simulink model "ss_ulinsys_itae_sim"  (Simulink 5.0)
settings: Solver=ode4  StartTime=0.0  StopTime=30  RelTol=1e-3  AbsTol=1e-6
values from neighbouring files (symbols this model uses):
  a = -0.7962    [ss_rapport_itae.m]    (also in ss_rapport_lqr.m; ss_rapport_lqr_tunet.m)
  b = -27.87    [ss_rapport_itae.m]    (also in ss_rapport_lqr.m; ss_rapport_lqr_tunet.m)
  K_itae_d = acker(sysd.a,sysd.b,pcd_itae)    [ss_rapport_itae.m]    (also in ss_rapport_lqr.m; ss_rapport_lqr_tunet.m)
  loopsysd = c2d(loopsys,Ts)    [ss_rapport_itae.m]    (also in ss_rapport_lqr.m; ss_rapport_lqr_tunet.m)
  Lr = (acker(loopsysd.a(2,2)',loopsysd.a(1,2)',estpoled))'    [ss_rapport_itae.m]    (also in ss_rapport_lqr.m; ss_rapport_lqr_tunet.m)
  Nbar = Nu + K_itae_d*Nx    [ss_rapport_itae.m]    (also in ss_rapport_lqr.m; ss_rapport_lqr_tunet.m = Nu + K_lqr_d*Nx)
  Ts = 1/50    (= 0.02)    [ss_rapport_itae.m]    (also in ss_rapport_lqr.m; ss_rapport_lqr_tunet.m)
undefined symbols (not defined in the file or in its folder): sigbuilder_block
libraries: simulink x1
settings Model: Creator=ubha02  LastModifiedBy=mikkel  ExtModeAutoUpdateStatusClock=off

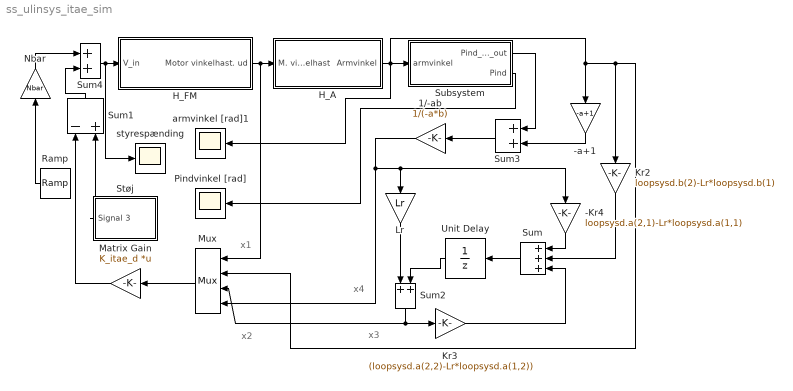
== system ss_ulinsys_itae_sim ==
  note: x4
  note: x3
  note: x2
  note: x1
  -Kr4 : Gain  Orientation=down  Gain=loopsysd.a(2,1)-Lr*loopsysd.a(1,1)  SaturateOnIntegerOverflow=on
  -a+1 : Gain  Orientation=down  Gain=-a+1  SaturateOnIntegerOverflow=on
  1/-ab : Gain  Orientation=left  Gain=1/(-a*b)  SaturateOnIntegerOverflow=on
  H_A : Subsystem
  H_FM : Subsystem
  Kr2 : Gain  Orientation=down  Gain=loopsysd.b(2)-Lr*loopsysd.b(1)  SaturateOnIntegerOverflow=on
  Kr3 : Gain  Gain=(loopsysd.a(2,2)-Lr*loopsysd.a(1,2))  SaturateOnIntegerOverflow=on
  Lr : Gain  Orientation=down  Gain=Lr  SaturateOnIntegerOverflow=on
  "Matrix Gain " : Gain  Orientation=left  Gain=K_itae_d  Multiplication=Matrix(K*u)  SaturateOnIntegerOverflow=on
  Mux : Mux  Orientation=left
  Nbar : Gain  Orientation=up  Gain=Nbar  SaturateOnIntegerOverflow=on
  Pindvinkel [rad] : Scope
      settings: SaveName=pindvinkel  DataFormat=Array
  Ramp : simulink/Sources/Ramp  Orientation=left  slope=0.02  start=0  X0=0
  Støj : Subsystem  Tag=STV Subsys  Orientation=left  StartFcn=sigbuilder_block('start');  StopFcn=sigbuilder_block('stop');  ClipboardFcn=sigbuilder_block('clipboard');  mask(Sigbuilder block){}
      mask help: Sigbuilder GUI
      mask init:
      | if ~strcmp(get_param(bdroot,'SimulationStatus'),'stopped') tuvar = sigbuilder_block('maskInit'); end
      settings: CopyFcn=sigbuilder_block('copy');  DeleteFcn=sigbuilder_block('delete');  ModelCloseFcn=sigbuilder_block('modelClose');  PreSaveFcn=sigbuilder_block('preSave');  NameChangeFcn=sigbuilder_block('namechange');  OpenFcn=sigbuilder_block('open',[50 50 520 400 ]);  CloseFcn=sigbuilder_block('close');
      mask Display: plot(0,0,100,100,[10,10,40,40,10],[80,20,20,80,80],[40,10],[50,50], [40,27,10],[65,72,56],[40,25,25,10],[28,28,43,43]);
  Subsystem : Subsystem
  Sum : Sum  Orientation=left  Inputs=+++  SaturateOnIntegerOverflow=on
  Sum1 : Sum  Orientation=up  Inputs=-+  SaturateOnIntegerOverflow=on
  Sum2 : Sum  Orientation=down  SaturateOnIntegerOverflow=on
  Sum3 : Sum  Orientation=left  SaturateOnIntegerOverflow=on
  Sum4 : Sum  SaturateOnIntegerOverflow=on
  Unit Delay : UnitDelay  Orientation=left  SampleTime=Ts
  armvinkel [rad]1 : Scope
      settings: SaveName=armvinkel  DataFormat=Array
  styrespænding : Scope
      settings: SaveName=styrespaending  DataFormat=Array
  wires:
  H_FM/1(Motor vinkelhast. ud) -> H_A/1(M. vinkelhast), Mux/1
  H_A/1(Armvinkel) -> armvinkel [rad]1/1, -a+1/1, Kr2/1, Mux/2, Subsystem/1(armvinkel)
  Subsystem/1(Pind_arm_out) -> Sum3/1
  Sum3/1 -> 1/-ab/1
  1/-ab/1 -> Lr/1, -Kr4/1, Mux/4
  -a+1/1 -> Sum3/2
  "Matrix Gain "/1 -> Sum1/1
  Sum/1 -> Unit Delay/1
  Unit Delay/1 -> Sum2/2
  Lr/1 -> Sum2/1
  Kr3/1 -> Sum/3
  Kr2/1 -> Sum/2
  -Kr4/1 -> Sum/1
  Sum2/1 -> Kr3/1, Mux/3
  Subsystem/2(Pind) -> Pindvinkel [rad]/1
  Mux/1 -> "Matrix Gain "/1
  Støj/1(Signal 3) -> Sum1/2
  Sum4/1 -> H_FM/1(V_in), styrespænding/1
  Sum1/1 -> Sum4/2
  Ramp/1 -> Nbar/1
  Nbar/1 -> Sum4/1

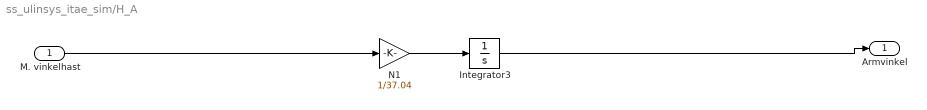
== system ss_ulinsys_itae_sim/H_A ==
  M. vinkelhast : Inport
  Integrator3 : Integrator
  N1 : Gain  Gain=1/37.04  SaturateOnIntegerOverflow=on
  Armvinkel : Outport
  wires:
  M. vinkelhast/1 -> N1/1
  N1/1 -> Integrator3/1
  Integrator3/1 -> Armvinkel/1

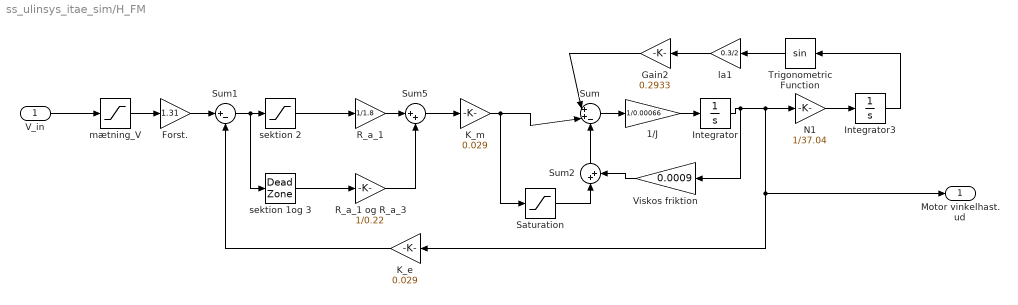
== system ss_ulinsys_itae_sim/H_FM ==
  V_in : Inport
  1/J : Gain  Gain=1/0.00066  SaturateOnIntegerOverflow=on
  Forst. : Gain  Gain=1.31  SaturateOnIntegerOverflow=on
  Gain2 : Gain  Orientation=left  Gain=0.2933  SaturateOnIntegerOverflow=on
  Integrator : Integrator
  Integrator3 : Integrator
  K_e : Gain  Orientation=left  Gain=0.029  SaturateOnIntegerOverflow=on
  K_m : Gain  Gain=0.029  SaturateOnIntegerOverflow=on
  N1 : Gain  Gain=1/37.04  SaturateOnIntegerOverflow=on
  R_a_1 : Gain  Gain=1/1.8  SaturateOnIntegerOverflow=on
  R_a_1 og R_a_3 : Gain  Gain=1/0.22  SaturateOnIntegerOverflow=on
  Saturation : Saturate  UpperLimit=0.3712  LowerLimit=-0.3712
  Sum : Sum  Inputs=|++-  SaturateOnIntegerOverflow=on
  Sum1 : Sum  Inputs=|+-  SaturateOnIntegerOverflow=on
  Sum2 : Sum  Orientation=up  Inputs=|++  SaturateOnIntegerOverflow=on
  Sum5 : Sum  Inputs=|++  SaturateOnIntegerOverflow=on
  Trigonometric Function : Trigonometry  Orientation=left
  Viskos friktion : Gain  Orientation=left  Gain=0.0009  SaturateOnIntegerOverflow=on
  la1 : Gain  Orientation=left  Gain=0.3/2  SaturateOnIntegerOverflow=on
  mætning_V : Saturate  UpperLimit=5  LowerLimit=-5
  sektion 1og 3 : DeadZone  LowerValue=-1  UpperValue=1  SaturateOnIntegerOverflow=on
  sektion 2 : Saturate  UpperLimit=1  LowerLimit=-1
  Motor vinkelhast. ud : Outport
  wires:
  V_in/1 -> mætning_V/1
  Forst./1 -> Sum1/1
  mætning_V/1 -> Forst./1
  Sum/1 -> 1/J/1
  1/J/1 -> Integrator/1
  Integrator/1 -> Viskos friktion/1, N1/1, K_e/1, Motor vinkelhast. ud/1
  sektion 1og 3/1 -> R_a_1 og R_a_3/1
  R_a_1/1 -> Sum5/1
  R_a_1 og R_a_3/1 -> Sum5/2
  Sum5/1 -> K_m/1
  sektion 2/1 -> R_a_1/1
  Sum1/1 -> sektion 2/1, sektion 1og 3/1
  K_e/1 -> Sum1/2
  N1/1 -> Integrator3/1
  la1/1 -> Gain2/1
  Gain2/1 -> Sum/1
  K_m/1 -> Sum/2, Saturation/1
  Sum2/1 -> Sum/3
  Viskos friktion/1 -> Sum2/2
  Saturation/1 -> Sum2/1
  Integrator3/1 -> Trigonometric Function/1
  Trigonometric Function/1 -> la1/1

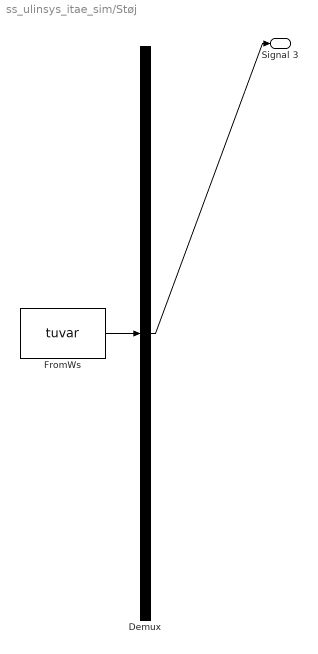
== system ss_ulinsys_itae_sim/Støj ==
  Demux : Demux  Tag=STV Demux  Outputs=1
  FromWs : FromWorkspace  Tag=STV FromWs  VariableName=tuvar  SampleTime=0  SigBuilderData=DataTag0
      SigBuilderData=|
      | channels.label = 'Signal 3'
      | channels.allXData = {[0 0.06 0.06 30]}
      | channels.allYData = {[5.54 5.54 0 0]}
      | dataSet.timeRange = [0 30]
      | dataSet.name = 'Group 1'
  Signal 3 : Outport  Tag=STV Outport
  wires:
  FromWs/1 -> Demux/1
  Demux/1 -> Signal 3/1

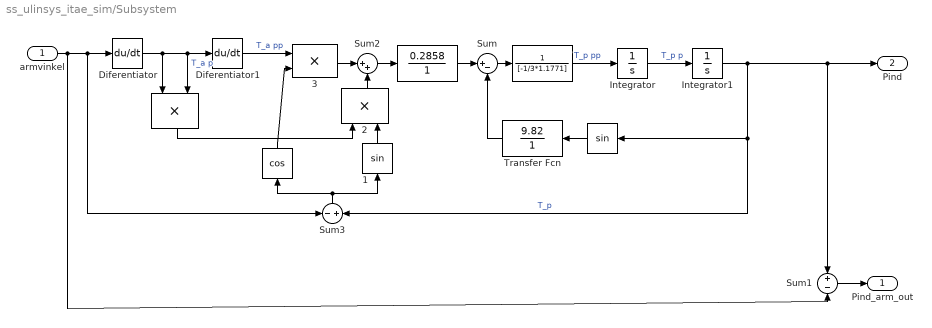
== system ss_ulinsys_itae_sim/Subsystem ==
  armvinkel : Inport
  " " : Trigonometry  Orientation=up  Operator=cos  OutputSignalType=real
  "  " : Product  Orientation=down  SaturateOnIntegerOverflow=on
  "    " : Trigonometry  Orientation=left  OutputSignalType=real
  "      " : TransferFcn  Denominator=[-1/3*1.1771]
  "        " : TransferFcn  Numerator=[0.2858]  Denominator=[1]
  " 1" : Trigonometry  Orientation=up  OutputSignalType=real
  " 2" : Product  Orientation=up  SaturateOnIntegerOverflow=on
  " 3" : Product  SaturateOnIntegerOverflow=on
  Diferentiator : Derivative
  Diferentiator1 : Derivative
  Integrator : Integrator
  Integrator1 : Integrator
  Sum : Sum  Inputs=|+-  SaturateOnIntegerOverflow=on
  Sum1 : Sum  Inputs=+-  SaturateOnIntegerOverflow=on
  Sum2 : Sum  Inputs=|++  SaturateOnIntegerOverflow=on
  Sum3 : Sum  Orientation=up  Inputs=-+  SaturateOnIntegerOverflow=on
  Transfer Fcn : TransferFcn  Orientation=left  Numerator=[9.82]  Denominator=[1]
  Pind_arm_out : Outport
  Pind : Outport  Port=2
  wires:
  Diferentiator/1 -> Diferentiator1/1, "  "/2, "  "/1  "T_a p"
  Diferentiator1/1 -> " 3"/1  "T_a pp"
  Integrator/1 -> Integrator1/1  "T_p p"
  "      "/1 -> Integrator/1  "T_p pp"
  Integrator1/1 -> "    "/1, Sum3/2, Sum1/1, Pind/1  "T_p"
  "    "/1 -> Transfer Fcn/1
  "        "/1 -> Sum/1
  Sum/1 -> "      "/1
  " "/1 -> " 3"/2
  Sum2/1 -> "        "/1
  " 3"/1 -> Sum2/1
  "  "/1 -> " 2"/1
  " 1"/1 -> " 2"/2
  " 2"/1 -> Sum2/2
  Sum3/1 -> " 1"/1, " "/1
  armvinkel/1 -> Diferentiator/1, Sum3/1, Sum1/2
  Transfer Fcn/1 -> Sum/2
  Sum1/1 -> Pind_arm_out/1
